simulink model "ReglareNivelbuclainchisaPID"  (R2024b)
settings: Solver=VariableStepAuto  StartTime=0.0  StopTime=1000  RelTol=1e-3
values from neighbouring files (symbols this model uses):
  A = 332.5    [scriptProiect.m]
  C = 9    [scriptProiect.m]
  h0 = 10.5    [scriptProiect.m]
  k = 0.035    [scriptProiect.m]
  k11 = k2^2 + 4*(k-k3)*k1    (= 0.0890826)    [scriptProiect.m]
  k12 = 8 * (k-k3)    (= 0.2848)    [scriptProiect.m]
  k13 = 2 * (k-k3)    (= 0.0712)    [scriptProiect.m]
  k2 = -0.015    [scriptProiect.m]
  keta = 8 * 10^-5    (= 8e-05)    [scriptProiect.m]
  KR = Tp/T0/kp    (= 2.40963855422)    [scriptProiect.m]
  q0 = 29.2    [scriptProiect.m]
  Rm = 3    [scriptProiect.m]
  Ti = Tp    (= 154)    [scriptProiect.m]
libraries: slpidlib x2
settings Model: Creator=Teo  LastModifiedBy=Teo

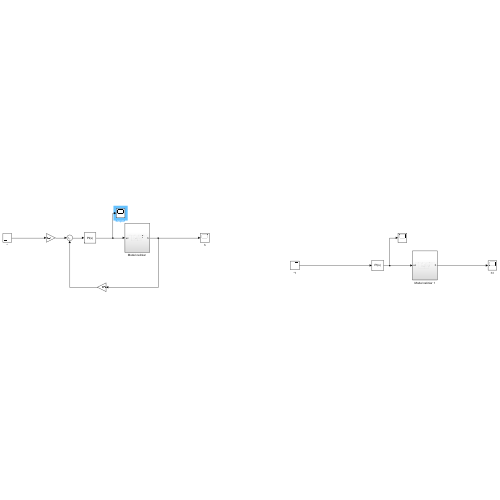
[thumbnail: Simulink's stored preview of the top-level diagram]
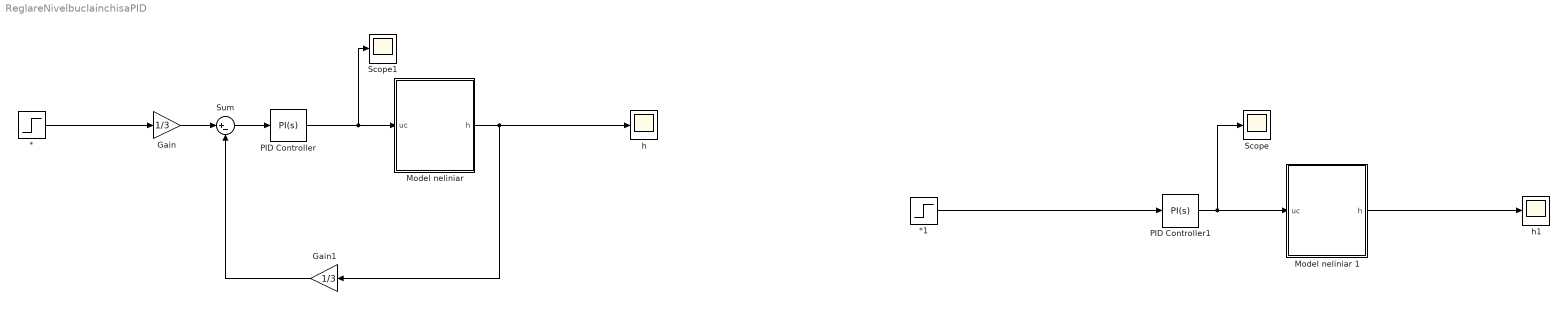
== system ReglareNivelbuclainchisaPID ==
  * : Step  Time=0  After=13  SampleTime=0
  *1 : Step  Time=0  After=13  SampleTime=0
  Gain : Gain  Gain=1/3
  Gain1 : Gain  Gain=1/3
  "Model neliniar " : Subsystem
  Model neliniar 1 : Subsystem
  PID Controller : slpidlib/PID Controller  Controller=PI  Form=Parallel  TimeDomain=Continuous-time  UseExternalTs=off  SampleTime=-1  IntegratorMethod=Forward Euler  FilterMethod=Forward Euler  ControllerParametersSource=internal  P=KR  I=KR/Ti  UseKiTs=off  D=0  UseExternalDerivativeSource=off  N=100  UseFilter=on  TunerSelectOption=Transfer Function Based (PID Tuner App)  InitialConditionSource=internal  InitialConditionForIntegrator=5  InitialConditionForFilter=0  DifferentiatorICPrevScaledInput=0  ExternalReset=none  TrackingMode=off  Kt=1  LimitOutput=off  SatLimitsSource=internal  UpperSaturationLimit=inf  LowerSaturationLimit=-inf  LinearizeAsGain=on  AntiWindupMode=none  Kb=1  LimitIntegrator=off  UpperIntegratorSaturationLimit=inf  LowerIntegratorSaturationLimit=-inf  POutMin=[]  POutMax=[]  IOutMin=[]  IOutMax=[]  DOutMin=[]  DOutMax=[]  NOutMin=[]  NOutMax=[]  SumOutMin=[]  SumOutMax=[]  SaturationOutMin=[]  SaturationOutMax=[]  PParamMin=[]  PParamMax=[]  IParamMin=[]  IParamMax=[]  DParamMin=[]  DParamMax=[]  NParamMin=[]  NParamMax=[]  KbParamMin=[]  KbParamMax=[]  KtParamMin=[]  KtParamMax=[]  KbOutMin=[]  KbOutMax=[]  KtOutMin=[]  KtOutMax=[]  IntegratorOutMin=[]  IntegratorOutMax=[]  FilterOutMin=[]  FilterOutMax=[]  SumI1OutMin=[]  SumI1OutMax=[]  SumI2OutMin=[]  SumI2OutMax=[]  SumI3OutMin=[]  SumI3OutMax=[]  SumI4OutMin=[]  SumI4OutMax=[]  SumDOutMin=[]  SumDOutMax=[]  DifferentiatorOutMin=[]  DifferentiatorOutMax=[]  FilterDiffOutCoefMin=[]  FilterDiffOutCoefMax=[]  ReciprocalOutMin=[]  ReciprocalOutMax=[]  SumDenOutMin=[]  SumDenOutMax=[]  SumNumOutMin=[]  SumNumOutMax=[]  DivideOutMin=[]  DivideOutMax=[]  UdiffTsProdOutMin=[]  UdiffTsProdOutMax=[]  NTsProdOutMin=[]  NTsProdOutMax=[]  UintegralTsProdOutMin=[]  UintegralTsProdOutMax=[]  UngainTsProdOutMin=[]  UngainTsProdOutMax=[]  ClampingZeroOutDataTypeStr=Inherit: Inherit via back propagation  ClampingZeroOutMin=[]  ClampingZeroOutMax=[]  FilterDenConstantOutDataTypeStr=Inherit: Inherit via back propagation  FilterDenConstantOutMin=[]  FilterDenConstantOutMax=[]  PCopyOutDataTypeStr=Inherit: Inherit via back propagation  PCopyOutMin=[]  PCopyOutMax=[]  NCopyOutDataTypeStr=Inherit: Inherit via back propagation  NCopyOutMin=[]  NCopyOutMax=[]  IntegratorContinuousStateAttributes=''  IntegratorStateMustResolveToSignalObject=off  IntegratorRTWStateStorageClass=Auto  FilterContinuousStateAttributes=''  FilterStateMustResolveToSignalObject=off  FilterRTWStateStorageClass=Auto  ParallelPVariant=InternalParameters  IdealPVariant=Disabled  IVariant=InternalParameters  DVariant=Disabled  IntegratorVariant=Continuous  SatVariant=Disabled  AWVariant=Passthrough  PCopyVariant=Disabled  TRVariant=Disabled  FdbkBlocksVariant=Forward  IdealPFdbkVariant=Disabled  SatFdbkVariant=Disabled  DerivativeFilterVariant=Disabled  NVariant=Disabled  NCopyVariant=Disabled_SignalSpec  FilterICVariant=Disabled  IntegratorICVariant=InternalICs  ExternalResetVariant=Disabled  TRSumVariant=Passthrough  SumFdbkVariant=Disabled  SumVariant=Sum_PI  TsampFilterVariant=InternalTs  TsampNgainVariant=Passthrough  TsampIntegralVariant=Disabled_SignalSpec  ExternalSaturationOutDataTypeStr=Inherit: Same as second input  DerivativeSourceVariant=Disabled  PreIntVariant=InternalPreInt
  PID Controller1 : slpidlib/PID Controller  Controller=PI  Form=Parallel  TimeDomain=Continuous-time  UseExternalTs=off  SampleTime=-1  IntegratorMethod=Forward Euler  FilterMethod=Forward Euler  ControllerParametersSource=internal  P=KR  I=KR/Ti  UseKiTs=off  D=0  UseExternalDerivativeSource=off  N=100  UseFilter=on  TunerSelectOption=Transfer Function Based (PID Tuner App)  InitialConditionSource=internal  InitialConditionForIntegrator=5  InitialConditionForFilter=0  DifferentiatorICPrevScaledInput=0  ExternalReset=none  TrackingMode=off  Kt=1  LimitOutput=off  SatLimitsSource=internal  UpperSaturationLimit=inf  LowerSaturationLimit=-inf  LinearizeAsGain=on  AntiWindupMode=none  Kb=1  LimitIntegrator=off  UpperIntegratorSaturationLimit=inf  LowerIntegratorSaturationLimit=-inf  POutMin=[]  POutMax=[]  IOutMin=[]  IOutMax=[]  DOutMin=[]  DOutMax=[]  NOutMin=[]  NOutMax=[]  SumOutMin=[]  SumOutMax=[]  SaturationOutMin=[]  SaturationOutMax=[]  PParamMin=[]  PParamMax=[]  IParamMin=[]  IParamMax=[]  DParamMin=[]  DParamMax=[]  NParamMin=[]  NParamMax=[]  KbParamMin=[]  KbParamMax=[]  KtParamMin=[]  KtParamMax=[]  KbOutMin=[]  KbOutMax=[]  KtOutMin=[]  KtOutMax=[]  IntegratorOutMin=[]  IntegratorOutMax=[]  FilterOutMin=[]  FilterOutMax=[]  SumI1OutMin=[]  SumI1OutMax=[]  SumI2OutMin=[]  SumI2OutMax=[]  SumI3OutMin=[]  SumI3OutMax=[]  SumI4OutMin=[]  SumI4OutMax=[]  SumDOutMin=[]  SumDOutMax=[]  DifferentiatorOutMin=[]  DifferentiatorOutMax=[]  FilterDiffOutCoefMin=[]  FilterDiffOutCoefMax=[]  ReciprocalOutMin=[]  ReciprocalOutMax=[]  SumDenOutMin=[]  SumDenOutMax=[]  SumNumOutMin=[]  SumNumOutMax=[]  DivideOutMin=[]  DivideOutMax=[]  UdiffTsProdOutMin=[]  UdiffTsProdOutMax=[]  NTsProdOutMin=[]  NTsProdOutMax=[]  UintegralTsProdOutMin=[]  UintegralTsProdOutMax=[]  UngainTsProdOutMin=[]  UngainTsProdOutMax=[]  ClampingZeroOutDataTypeStr=Inherit: Inherit via back propagation  ClampingZeroOutMin=[]  ClampingZeroOutMax=[]  FilterDenConstantOutDataTypeStr=Inherit: Inherit via back propagation  FilterDenConstantOutMin=[]  FilterDenConstantOutMax=[]  PCopyOutDataTypeStr=Inherit: Inherit via back propagation  PCopyOutMin=[]  PCopyOutMax=[]  NCopyOutDataTypeStr=Inherit: Inherit via back propagation  NCopyOutMin=[]  NCopyOutMax=[]  IntegratorContinuousStateAttributes=''  IntegratorStateMustResolveToSignalObject=off  IntegratorRTWStateStorageClass=Auto  FilterContinuousStateAttributes=''  FilterStateMustResolveToSignalObject=off  FilterRTWStateStorageClass=Auto  ParallelPVariant=InternalParameters  IdealPVariant=Disabled  IVariant=InternalParameters  DVariant=Disabled  IntegratorVariant=Continuous  SatVariant=Disabled  AWVariant=Passthrough  PCopyVariant=Disabled  TRVariant=Disabled  FdbkBlocksVariant=Forward  IdealPFdbkVariant=Disabled  SatFdbkVariant=Disabled  DerivativeFilterVariant=Disabled  NVariant=Disabled  NCopyVariant=Disabled_SignalSpec  FilterICVariant=Disabled  IntegratorICVariant=InternalICs  ExternalResetVariant=Disabled  TRSumVariant=Passthrough  SumFdbkVariant=Disabled  SumVariant=Sum_PI  TsampFilterVariant=InternalTs  TsampNgainVariant=Passthrough  TsampIntegralVariant=Disabled_SignalSpec  ExternalSaturationOutDataTypeStr=Inherit: Same as second input  DerivativeSourceVariant=Disabled  PreIntVariant=InternalPreInt
  Scope : Scope
  Scope1 : Scope
  Sum : Sum  Inputs=|+-
  h : Scope
  h1 : Scope
  wires:
  */1 -> Gain/1
  PID Controller/1 -> Scope1/1, "Model neliniar "/1(uc)
  Gain1/1 -> Sum/2
  Gain/1 -> Sum/1
  "Model neliniar "/1(h) -> h/1, Gain1/1
  Sum/1 -> PID Controller/1
  PID Controller1/1 -> Scope/1, Model neliniar 1/1(uc)
  Model neliniar 1/1(h) -> h1/1
  *1/1 -> PID Controller1/1

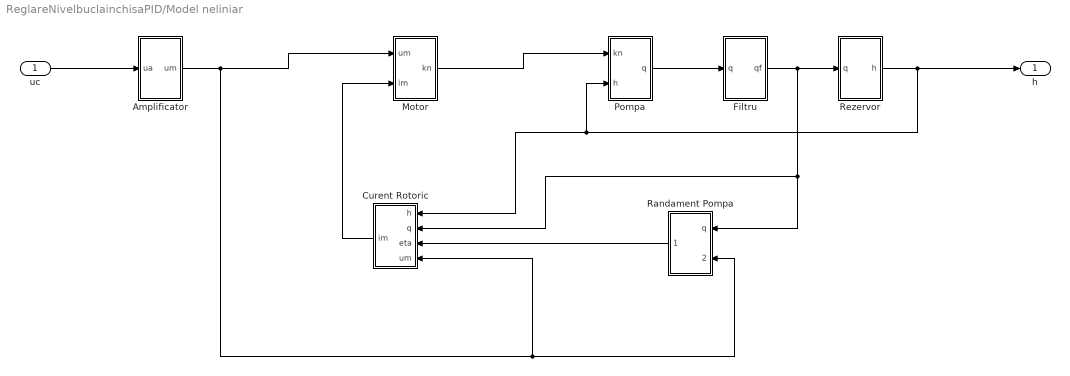
== system ReglareNivelbuclainchisaPID/Model neliniar  ==
  uc : Inport
  Amplificator : Subsystem
  Curent Rotoric : Subsystem
  Filtru : Subsystem
  Motor : Subsystem
  Pompa : Subsystem
  Randament Pompa : Subsystem
  Rezervor : Subsystem
  h : Outport
  wires:
  Curent Rotoric/1(im) -> Motor/2(im)
  Randament Pompa/1(eta) -> Curent Rotoric/3(eta)
  Motor/1(kn) -> Pompa/1(kn)
  Rezervor/1(h) -> h/1, Curent Rotoric/1(h), Pompa/2(h)
  Filtru/1(qf) -> Randament Pompa/1(q), Curent Rotoric/2(q), Rezervor/1(q)
  Pompa/1(q) -> Filtru/1(q)
  uc/1 -> Amplificator/1(ua)
  Amplificator/1(um) -> Randament Pompa/2(um), Curent Rotoric/4(um), Motor/1(um)

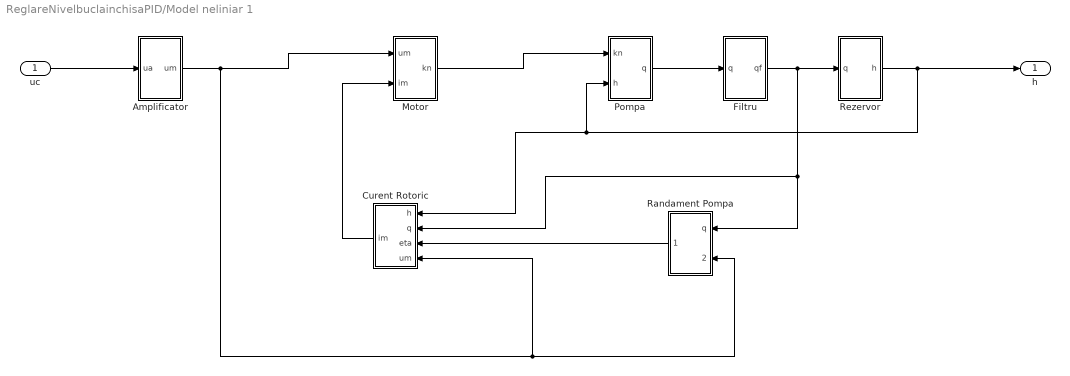
== system ReglareNivelbuclainchisaPID/Model neliniar 1 ==
  uc : Inport
  Amplificator : Subsystem
  Curent Rotoric : Subsystem
  Filtru : Subsystem
  Motor : Subsystem
  Pompa : Subsystem
  Randament Pompa : Subsystem
  Rezervor : Subsystem
  h : Outport
  wires:
  Curent Rotoric/1(im) -> Motor/2(im)
  Randament Pompa/1(eta) -> Curent Rotoric/3(eta)
  Motor/1(kn) -> Pompa/1(kn)
  Rezervor/1(h) -> h/1, Curent Rotoric/1(h), Pompa/2(h)
  Filtru/1(qf) -> Randament Pompa/1(q), Curent Rotoric/2(q), Rezervor/1(q)
  Pompa/1(q) -> Filtru/1(q)
  uc/1 -> Amplificator/1(ua)
  Amplificator/1(um) -> Randament Pompa/2(um), Curent Rotoric/4(um), Motor/1(um)

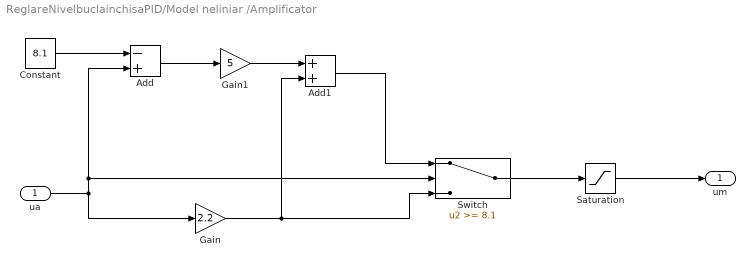
== system ReglareNivelbuclainchisaPID/Model neliniar /Amplificator ==
  ua : Inport
  Add : Sum  Inputs=-+
  Add1 : Sum
  Constant : Constant  Value=8.1
  Gain : Gain  Gain=2.2
  Gain1 : Gain  Gain=5
  Saturation : Saturate  UpperLimit=22  LowerLimit=0
  Switch : Switch  Threshold=8.1  SaturateOnIntegerOverflow=off  InputSameDT=off
  um : Outport
  wires:
  Add/1 -> Gain1/1
  Add1/1 -> Switch/1
  Switch/1 -> Saturation/1
  Constant/1 -> Add/1
  Saturation/1 -> um/1
  Gain/1 -> Switch/3, Add1/2
  ua/1 -> Add/2, Switch/2, Gain/1
  Gain1/1 -> Add1/1

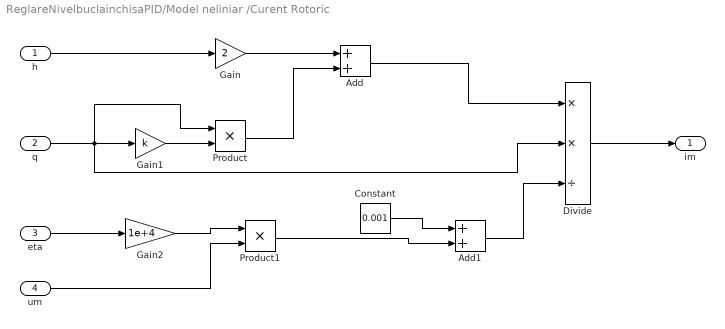
== system ReglareNivelbuclainchisaPID/Model neliniar /Curent Rotoric ==
  h : Inport
  q : Inport  Port=2
  eta : Inport  Port=3
  um : Inport  Port=4
  Add : Sum
  Add1 : Sum
  Constant : Constant  Value=0.001
  Divide : Product  Inputs=**/
  Gain : Gain  Gain=2
  Gain1 : Gain  Gain=k
  Gain2 : Gain  Gain=1e+4
  Product : Product
  Product1 : Product
  im : Outport
  wires:
  Gain1/1 -> Product/2
  Gain/1 -> Add/1
  Gain2/1 -> Product1/1
  q/1 -> Divide/2, Product/1, Gain1/1
  Add1/1 -> Divide/3
  Product1/1 -> Add1/2
  um/1 -> Product1/2
  Add/1 -> Divide/1
  Product/1 -> Add/2
  eta/1 -> Gain2/1
  h/1 -> Gain/1
  Constant/1 -> Add1/1
  Divide/1 -> im/1

== system ReglareNivelbuclainchisaPID/Model neliniar /Filtru ==
  q : Inport
  Integrator : Integrator  InitialCondition=q0
  Sum : Sum  Inputs=|+-
  qf : Outport
  wires:
  q/1 -> Sum/1
  Integrator/1 -> qf/1, Sum/2
  Sum/1 -> Integrator/1

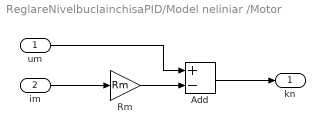
== system ReglareNivelbuclainchisaPID/Model neliniar /Motor ==
  um : Inport
  im : Inport  Port=2
  Add : Sum  Inputs=+-
  Rm : Gain  Gain=Rm
  kn : Outport
  wires:
  im/1 -> Rm/1
  Rm/1 -> Add/2
  um/1 -> Add/1
  Add/1 -> kn/1

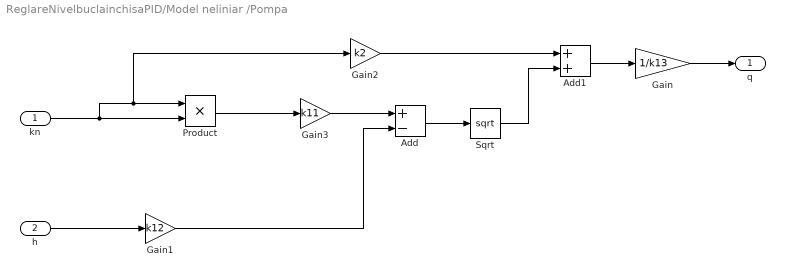
== system ReglareNivelbuclainchisaPID/Model neliniar /Pompa ==
  kn : Inport
  h : Inport  Port=2
  Add : Sum  Inputs=+-
  Add1 : Sum
  Gain : Gain  Gain=1/k13
  Gain1 : Gain  Gain=k12
  Gain2 : Gain  Gain=k2
  Gain3 : Gain  Gain=k11
  Product : Product
  Sqrt : Sqrt
  q : Outport
  wires:
  Gain1/1 -> Add/2
  h/1 -> Gain1/1
  Sqrt/1 -> Add1/2
  Add1/1 -> Gain/1
  Gain3/1 -> Add/1
  Add/1 -> Sqrt/1
  Product/1 -> Gain3/1
  Gain/1 -> q/1
  Gain2/1 -> Add1/1
  kn/1 -> Gain2/1, Product/1, Product/2

== system ReglareNivelbuclainchisaPID/Model neliniar /Randament Pompa ==
  q : Inport
  um : Inport  Port=2
  Gain : Gain  Gain=keta
  Product : Product
  eta : Outport
  wires:
  um/1 -> Gain/1
  Product/1 -> eta/1
  Gain/1 -> Product/2
  q/1 -> Product/1

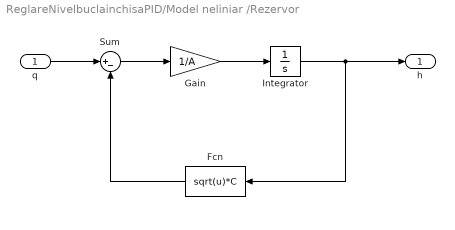
== system ReglareNivelbuclainchisaPID/Model neliniar /Rezervor ==
  q : Inport
  Fcn : Fcn  Expr=sqrt(u)*C
  Gain : Gain  Gain=1/A
  Integrator : Integrator  InitialCondition=h0
  Sum : Sum  Inputs=|+-
  h : Outport
  wires:
  Fcn/1 -> Sum/2
  Gain/1 -> Integrator/1
  Sum/1 -> Gain/1
  Integrator/1 -> h/1, Fcn/1
  q/1 -> Sum/1

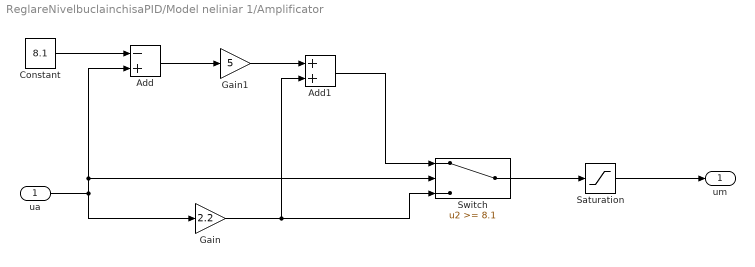
== system ReglareNivelbuclainchisaPID/Model neliniar 1/Amplificator ==
  ua : Inport
  Add : Sum  Inputs=-+
  Add1 : Sum
  Constant : Constant  Value=8.1
  Gain : Gain  Gain=2.2
  Gain1 : Gain  Gain=5
  Saturation : Saturate  UpperLimit=22  LowerLimit=0
  Switch : Switch  Threshold=8.1  SaturateOnIntegerOverflow=off  InputSameDT=off
  um : Outport
  wires:
  Add/1 -> Gain1/1
  Add1/1 -> Switch/1
  Switch/1 -> Saturation/1
  Constant/1 -> Add/1
  Saturation/1 -> um/1
  Gain/1 -> Switch/3, Add1/2
  ua/1 -> Add/2, Switch/2, Gain/1
  Gain1/1 -> Add1/1

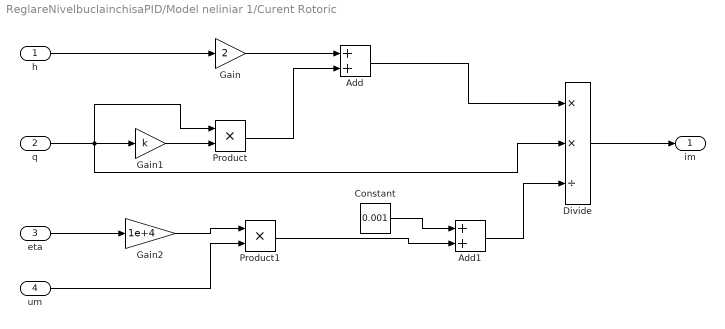
== system ReglareNivelbuclainchisaPID/Model neliniar 1/Curent Rotoric ==
  h : Inport
  q : Inport  Port=2
  eta : Inport  Port=3
  um : Inport  Port=4
  Add : Sum
  Add1 : Sum
  Constant : Constant  Value=0.001
  Divide : Product  Inputs=**/
  Gain : Gain  Gain=2
  Gain1 : Gain  Gain=k
  Gain2 : Gain  Gain=1e+4
  Product : Product
  Product1 : Product
  im : Outport
  wires:
  Gain1/1 -> Product/2
  Gain/1 -> Add/1
  Gain2/1 -> Product1/1
  q/1 -> Divide/2, Product/1, Gain1/1
  Add1/1 -> Divide/3
  Product1/1 -> Add1/2
  um/1 -> Product1/2
  Add/1 -> Divide/1
  Product/1 -> Add/2
  eta/1 -> Gain2/1
  h/1 -> Gain/1
  Constant/1 -> Add1/1
  Divide/1 -> im/1

== system ReglareNivelbuclainchisaPID/Model neliniar 1/Filtru ==
  q : Inport
  Integrator : Integrator  InitialCondition=q0
  Sum : Sum  Inputs=|+-
  qf : Outport
  wires:
  q/1 -> Sum/1
  Integrator/1 -> qf/1, Sum/2
  Sum/1 -> Integrator/1

== system ReglareNivelbuclainchisaPID/Model neliniar 1/Motor ==
  um : Inport
  im : Inport  Port=2
  Add : Sum  Inputs=+-
  Rm : Gain  Gain=Rm
  kn : Outport
  wires:
  im/1 -> Rm/1
  Rm/1 -> Add/2
  um/1 -> Add/1
  Add/1 -> kn/1

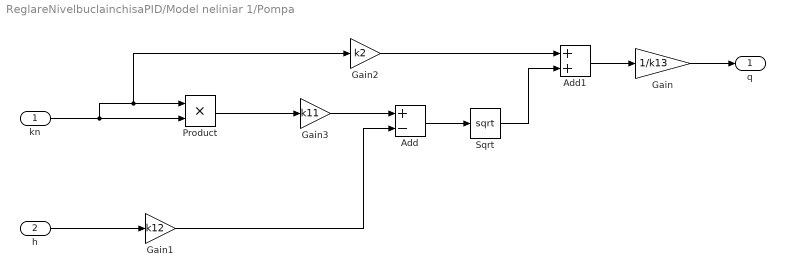
== system ReglareNivelbuclainchisaPID/Model neliniar 1/Pompa ==
  kn : Inport
  h : Inport  Port=2
  Add : Sum  Inputs=+-
  Add1 : Sum
  Gain : Gain  Gain=1/k13
  Gain1 : Gain  Gain=k12
  Gain2 : Gain  Gain=k2
  Gain3 : Gain  Gain=k11
  Product : Product
  Sqrt : Sqrt
  q : Outport
  wires:
  Gain1/1 -> Add/2
  h/1 -> Gain1/1
  Sqrt/1 -> Add1/2
  Add1/1 -> Gain/1
  Gain3/1 -> Add/1
  Add/1 -> Sqrt/1
  Product/1 -> Gain3/1
  Gain/1 -> q/1
  Gain2/1 -> Add1/1
  kn/1 -> Gain2/1, Product/1, Product/2

== system ReglareNivelbuclainchisaPID/Model neliniar 1/Randament Pompa ==
  q : Inport
  um : Inport  Port=2
  Gain : Gain  Gain=keta
  Product : Product
  eta : Outport
  wires:
  um/1 -> Gain/1
  Product/1 -> eta/1
  Gain/1 -> Product/2
  q/1 -> Product/1

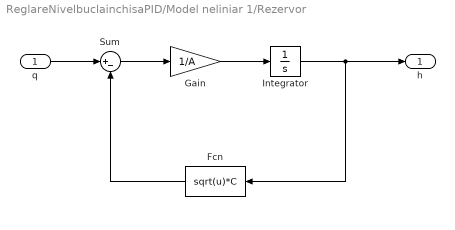
== system ReglareNivelbuclainchisaPID/Model neliniar 1/Rezervor ==
  q : Inport
  Fcn : Fcn  Expr=sqrt(u)*C
  Gain : Gain  Gain=1/A
  Integrator : Integrator  InitialCondition=h0
  Sum : Sum  Inputs=|+-
  h : Outport
  wires:
  Fcn/1 -> Sum/2
  Gain/1 -> Integrator/1
  Sum/1 -> Gain/1
  Integrator/1 -> h/1, Fcn/1
  q/1 -> Sum/1
